simulink library "MPC_51_v0_CL"  (R2020a)
settings: Solver=VariableStepAuto  StartTime=0.0  StopTime=10.0  RelTol=1e-3
undefined symbols (not defined in the file): Int, sig_info, UNCC
libraries: MPC_Sublibraries x3
settings Model: Creator=John Jr  LastModifiedBy=John Jr
settings DataIOCC: ReturnWorkspaceOutputs=off
settings DebuggingCC: ArithmeticOperatorsInVariantConditions=warning
settings SFSimCC: CustomCodeUndefinedFunction=UseInterfaceOnly

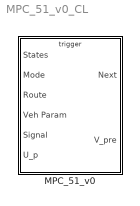
== system MPC_51_v0_CL ==
  MPC_51_v0 : Subsystem  TreatAsAtomicUnit=on
      mask Display:
      | patch([0 1 1 0], [0 0 1 1],[1 .8 1])
      | 
      | port_label('input',1,'\fontname{Cambria Math}States','texmode','on')
      | port_label('input',2,'\fontname{Cambria Math}Mode','texmode','on')
      | port_label('input',3,'\fontname{Cambria Math}Route','texmode','on')
      | port_label('input',4,'\fontname{Cambria Math}Param','texmode','on')
      | port_label('input',5,'\fontname{Cambria Math}Signal','texmode','on')
      | port_label('input',6,'\fontname{Cambria Math}T_{prev}','texmode','on')
      | 
      | port_label('output',1,'\fontname{Cambria Math}V_{MPC},T_{MPC}','texmode','on')
      | port_label('output',2,'\fontname{Cambria Math}V_{des}(1)','texmode','on')
      | 
      | port_label('trigger','\spadesuit','texmode','on')
      | 
      | disp('\fontname{Cambria Math}\fontsize{12}  MPC v0\newline  51 Step','texmode','on')

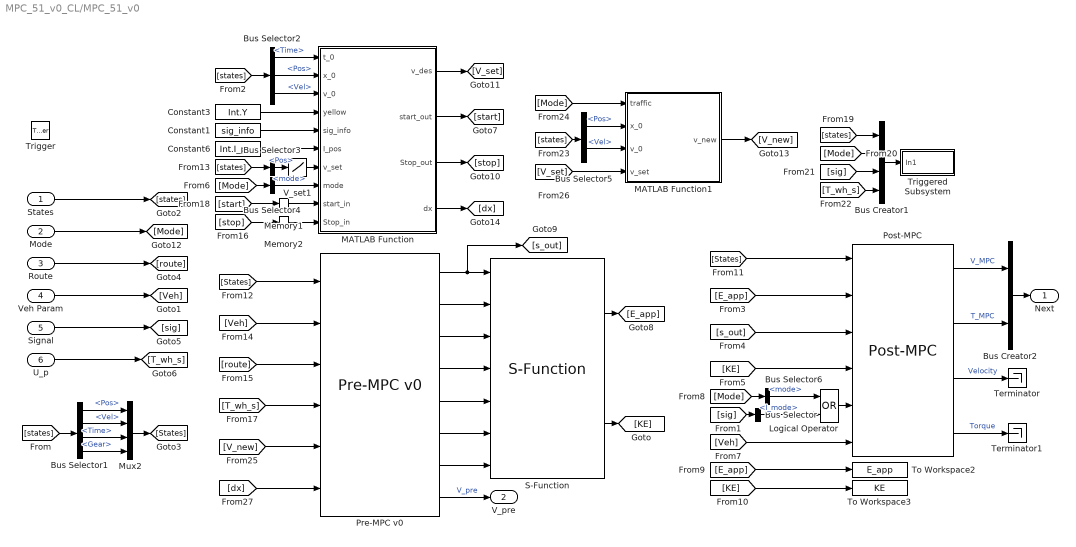
== system MPC_51_v0_CL/MPC_51_v0 ==
  States : Inport
  Mode : Inport  Port=2
  Route : Inport  Port=3
  Veh Param : Inport  Port=4
  Signal : Inport  Port=5
  U_p : Inport  Port=6
  Trigger : TriggerPort  TriggerType=falling  VariantControl=Variant
  Bus Creator1 : BusCreator  Inputs=4
  Bus Creator2 : BusCreator  Inputs=2
  Bus Selector : BusSelector  OutputSignals=I_mode
  Bus Selector1 : BusSelector  OutputSignals=Pos,Vel,Time,Gear
  Bus Selector2 : BusSelector  OutputSignals=Time,Pos,Vel
  Bus Selector3 : BusSelector  OutputSignals=Pos
  Bus Selector4 : BusSelector  OutputSignals=mode
  Bus Selector5 : BusSelector  OutputSignals=Pos,Vel
  Bus Selector6 : BusSelector  OutputSignals=mode
  Constant1 : Constant  Value=sig_info
  Constant3 : Constant  Value=Int.Y
  Constant6 : Constant  Value=Int.I_pos
  Logical Operator : Logic  Operator=OR  AllPortsSameDT=off  OutDataTypeStr=boolean
  MATLAB Function : MATLAB Function  TreatAsAtomicUnit=on
  MATLAB Function1 : MATLAB Function  TreatAsAtomicUnit=on
  Memory1 : Memory  InitialCondition=[0 0]  InheritSampleTime=on
  Memory2 : Memory  InheritSampleTime=on
  Mux2 : Mux
  Post-MPC : MPC_Sublibraries/Post-MPC  SystemSampleTime=-1  Latency=0  AutoFrameSizeCalculation=off
  Pre-MPC v0 : MPC_Sublibraries/Pre-MPC v0  SystemSampleTime=-1  Latency=0  AutoFrameSizeCalculation=off
  S-Function : MPC_Sublibraries/S-Function  SFunctionModules=solver_51_v2_wrapper
  Terminator : Terminator
  Terminator1 : Terminator
  To Workspace2 : ToWorkspace  VariableName=E_app  SampleTime=-1
  To Workspace3 : ToWorkspace  VariableName=KE  SampleTime=-1
  Triggered Subsystem : Subsystem  TreatAsAtomicUnit=on
      mask Display:
      | patch([0 1 1 0], [0 0 1 1],[.8 1 .8])
      | 
      | port_label('input',1,'MPC input')
  V_set1 : Lookup_n-D  NumberOfTableDimensions=1  BreakpointsForDimension1=UNCC.X_vec  Table=UNCC.V_lim  InterpMethod=Flat  ExtrapMethod=Clip  InputSameDT=on
  Next : Outport  VectorParamsAs1DForOutWhenUnconnected=off
  V_pre : Outport  Port=2  VectorParamsAs1DForOutWhenUnconnected=off
  wires:
  Bus Selector/1 -> Logical Operator/2  "<I_mode>"
  [sig] -> Bus Selector/1
  States/1 -> [states]
  Route/1 -> [route]
  Bus Selector1/4 -> Mux2/4  "<Gear>"
  Bus Selector1/2 -> Mux2/2  "<Vel>"
  Bus Selector1/3 -> Mux2/3  "<Time>"
  Bus Selector1/1 -> Mux2/1  "<Pos>"
  [states] -> Bus Selector1/1
  Veh Param/1 -> [Veh]
  [Veh] -> Post-MPC/6
  Post-MPC/4 -> Terminator1/1  "Torque"
  Post-MPC/3 -> Terminator/1  "Velocity"
  Mux2/1 -> [States]
  [States] -> Post-MPC/1
  Mode/1 -> [Mode]
  [E_app] -> Post-MPC/2
  [s_out] -> Post-MPC/3
  [KE] -> Post-MPC/4
  Logical Operator/1 -> Post-MPC/5
  S-Function/2 -> [KE]
  S-Function/1 -> [E_app]
  Bus Creator2/1 -> Next/1
  Post-MPC/1 -> Bus Creator2/1  "V_MPC"
  Post-MPC/2 -> Bus Creator2/2  "T_MPC"
  Signal/1 -> [sig]
  [states] -> Bus Creator1/1
  [sig] -> Bus Creator1/3
  [T_wh_s] -> Bus Creator1/4
  Bus Creator1/1 -> Triggered Subsystem/1(In1)
  [Mode] -> Bus Creator1/2
  [KE] -> To Workspace3/1
  [E_app] -> To Workspace2/1
  [T_wh_s] -> Pre-MPC v0/4
  [route] -> Pre-MPC v0/3
  [Veh] -> Pre-MPC v0/2
  [States] -> Pre-MPC v0/1
  Pre-MPC v0/1 -> S-Function/1, [s_out]
  Pre-MPC v0/2 -> S-Function/2
  Pre-MPC v0/3 -> S-Function/3
  Pre-MPC v0/4 -> S-Function/4
  Pre-MPC v0/5 -> S-Function/5
  Pre-MPC v0/6 -> S-Function/6
  Pre-MPC v0/7 -> S-Function/7
  Pre-MPC v0/8 -> V_pre/1  "V_pre"
  U_p/1 -> [T_wh_s]
  [states] -> Bus Selector2/1
  Bus Selector2/3 -> MATLAB Function/3(v_0)  "<Vel>"
  Bus Selector2/2 -> MATLAB Function/2(x_0)  "<Pos>"
  Bus Selector2/1 -> MATLAB Function/1(t_0)  "<Time>"
  Constant6/1 -> MATLAB Function/6(I_pos)
  Constant1/1 -> MATLAB Function/5(sig_info)
  Constant3/1 -> MATLAB Function/4(yellow)
  [stop] -> Memory2/1
  [start] -> Memory1/1
  Memory1/1 -> MATLAB Function/9(start_in)
  Memory2/1 -> MATLAB Function/10(Stop_in)
  MATLAB Function/2(start_out) -> [start]
  MATLAB Function/3(Stop_out) -> [stop]
  [states] -> Bus Selector3/1
  [Mode] -> Bus Selector4/1
  Bus Selector4/1 -> MATLAB Function/8(mode)  "<mode>"
  MATLAB Function/1(v_des) -> [V_set]
  [V_set] -> MATLAB Function1/4(v_set)
  Bus Selector5/1 -> MATLAB Function1/2(x_0)  "<Pos>"
  [Mode] -> MATLAB Function1/1(traffic)
  Bus Selector5/2 -> MATLAB Function1/3(v_0)  "<Vel>"
  [states] -> Bus Selector5/1
  MATLAB Function1/1(v_new) -> [V_new]
  [V_new] -> Pre-MPC v0/5
  [Mode] -> Bus Selector6/1
  Bus Selector6/1 -> Logical Operator/1  "<mode>"
  MATLAB Function/4(dx) -> [dx]
  [dx] -> Pre-MPC v0/6
  V_set1/1 -> MATLAB Function/7(v_set)
  Bus Selector3/1 -> V_set1/1  "<Pos>"

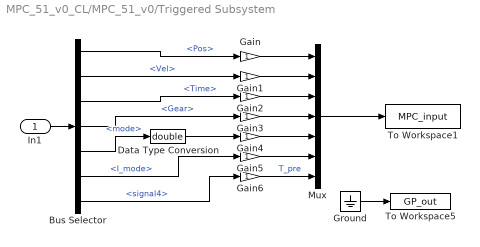
== system MPC_51_v0_CL/MPC_51_v0/Triggered Subsystem ==
  In1 : Inport
  Bus Selector : BusSelector  OutputSignals=signal1.Pos,signal1.Vel,signal1.Time,signal1.Gear,Traffic.mode,signal3.I_mode,signal4
  Data Type Conversion : DataTypeConversion  OutDataTypeStr=double
  Gain{,1..6} (7 alike) : Gain
  Ground : Ground
  Mux : Mux  Inputs=7
  To Workspace1 : ToWorkspace  VariableName=MPC_input  SaveFormat=Structure With Time  SampleTime=-1
  To Workspace5 : ToWorkspace  VariableName=GP_out  SampleTime=-1
  wires:
  Ground/1 -> To Workspace5/1
  In1/1 -> Bus Selector/1
  Bus Selector/1 -> Gain/1  "<Pos>"
  Bus Selector/6 -> Gain5/1  "<I_mode>"
  Bus Selector/5 -> Data Type Conversion/1  "<mode>"
  Bus Selector/4 -> Gain3/1  "<Gear>"
  Bus Selector/3 -> Gain2/1  "<Time>"
  Bus Selector/2 -> Gain1/1  "<Vel>"
  Bus Selector/7 -> Gain6/1  "<signal4>"
  Gain6/1 -> Mux/7  "T_pre"
  Gain5/1 -> Mux/6
  Gain4/1 -> Mux/5
  Gain3/1 -> Mux/4
  Gain2/1 -> Mux/3
  Gain1/1 -> Mux/2
  Gain/1 -> Mux/1
  Mux/1 -> To Workspace1/1
  Data Type Conversion/1 -> Gain4/1

== matlab function MPC_51_v0_CL/MPC_51_v0/MATLAB Function1 ==
  data: traffic input; v_new output; x_0 input; v_0 input; v_set input
function v_new  = fcn(traffic,x_0,v_0,v_set)

tau = 0.75;                 %   s - Driver reaction time
a_n = 2;                    %   m/s^2 - Maximum acceleration
b_n = -2*a_n;               %   m/s^2 - Maximum brake acceleration
b_hat = -2;                 %   m/s^2 - Estimated lead vehicle brake acceleration
t_n = 2;                    %   s - Safe following time

x_lead = traffic(1);        %   m - Lead vehicle poaition
v_lead = traffic(2);        %   m/s - Lead vehicle velocity
s_n = max(v_lead*t_n,5);    %   m - Safe following distance
v_0 = max(v_0,0);

if x_lead-x_0 <= 0          %   Condition to prevent negative radical
    x_lead = x_0;
    v_lead = v_0;
end

if traffic(4) == 0        %   In traffic?
    v_new = v_set;
else
    if (b_n^2*tau^2-b_n*(2*(x_lead-s_n-x_0)-v_0*tau-v_lead^2/b_hat)) > 0
        v_new = min(v_0+2.5*a_n*tau*(1-v_0/v_set)*sqrt(.025+v_0/v_set),...
            b_n*tau+sqrt(b_n^2*tau^2-b_n*(2*(x_lead-s_n-x_0)-v_0*tau-v_lead^2/b_hat)));
    else
        v_new = 0;
    end
    v_new = max(v_new,0);
end

== matlab function MPC_51_v0_CL/MPC_51_v0/MATLAB Function ==
  data: t_0 input; v_des output; x_0 input; v_0 input; yellow input; sig_info input; I_pos input; v_set input; mode input; start_in input; Stop_in input; start_out output; Stop_out output; dx output
function [v_des,start_out,Stop_out,dx] = fcn(t_0,x_0,v_0,yellow,sig_info,I_pos,v_set,mode,start_in,Stop_in)

G = sig_info(:,:,2);                                    %   s - Intersection green phases 
Cs = sig_info(:,:,3);                                   %   s - Cycle start times 
window = 250;                                           %   m - Driver sight range
dt = .01;                                               %   s - Sample time
Idx1 = find(x_0-I_pos < 0,1,'first');                   %   Next upcoming intersection 
if isempty(Idx1)
    dx = 500;
else
    dx = I_pos(Idx1(1))-x_0;                            %   m - Distance to upcoming intersection 
end
if dx >= window
    Int_approach = 0;                                   %   No upcoming intersection 
else
    Int_approach = 1;                                   %   There is an upcoming intersection 
end
if Int_approach == 1
    Idx2 = find(Cs(Idx1(1),:) <= t_0,1,'last');         %   Current cycle # for upcoming intersection
    x_approach = v_0*yellow(Idx1(1));                            %   m - Distance to make yellow
    if t_0 < Cs(Idx1(1),Idx2(1))+G(Idx1(1),Idx2(1))-yellow(Idx1(1))
        light = 0;                                      %   Light is green
    elseif t_0 >= Cs(Idx1(1),Idx2(1))+G(Idx1(1),Idx2(1))-yellow(Idx1(1))...
            && t_0 < Cs(Idx1(1),Idx2(1))+G(Idx1(1),Idx2(1))
        light = 1;                                      %   Light is yellow
    else
        light = 2;                                      %   Light is red
    end
    if light == 0 && Stop_in == 1
        Stop_out = 0;
        start_in = [0 0];
    elseif (light == 1 && dx > x_approach) || light == 2 ...
            || (light == 1 && Stop_in == 1)
        Stop_out = 1;
        start_in = start_in';
    else
        Stop_out = 0;
        start_in = [0 0];
    end
else
    Stop_out = 0;
    start_in = [0 0];
end
if Stop_out == 1 && start_in(1) == 0
    start_in = [x_0,v_0];
end
if Stop_out == 1
    if mode == 1
        x_stop = linspace(start_in(1),I_pos(Idx1(1))-15,100);
    else
        x_stop = linspace(start_in(1),I_pos(Idx1(1))-5,100);
    end
    v_stop = linspace(start_in(2),0,100);
    v_des = interp1(x_stop,v_stop,x_0,'linear',0);
else
    v_des = v_set;
end
start_out = start_in;
end
